simulink model "p3_a"  (R2021b)
settings: Solver=VariableStepAuto  StartTime=0.0  StopTime=2.5  RelTol=1e-3
settings Model: Creator=mluser  LastModifiedBy=mluser

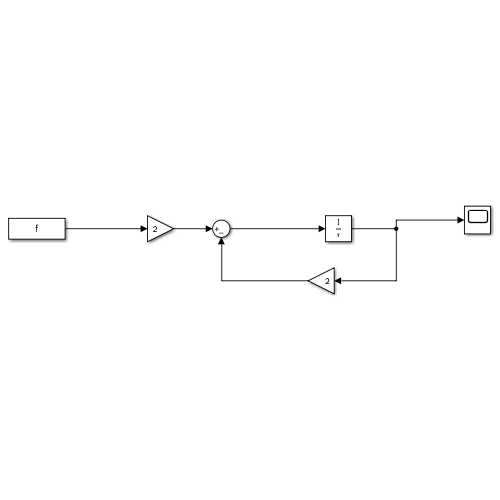
[thumbnail: Simulink's stored preview of the top-level diagram]
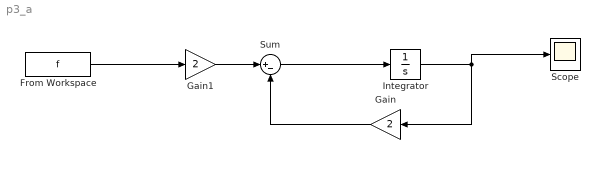
== system p3_a ==
  From Workspace : FromWorkspace  VariableName=f
  Gain : Gain  Gain=2
  Gain1 : Gain  Gain=2
  Integrator : Integrator
  Scope : Scope
  Sum : Sum  Inputs=|+-
  wires:
  Sum/1 -> Integrator/1
  Integrator/1 -> Scope/1, Gain/1
  Gain1/1 -> Sum/1
  Gain/1 -> Sum/2
  From Workspace/1 -> Gain1/1
